simulink model "basic_dynamic_ant"  (R2022a)
settings: Solver=VariableStepAuto  StartTime=0.0  StopTime=10.0  RelTol=1e-3
values from neighbouring files (symbols this model uses):
  configSequence = [robot.Bodies{4}.Joint.PositionLimits; -robot.Bodies{7}.Joint.PositionLimits]    [ant_grasp_only.m]
  dq0 = zeros(size(q0))    [ant_grasp_only.m]
  q0 = homeConfiguration(robot)    [ant_grasp_only.m]
  widgetDimensions = [0.2 0.02 0.07]    [ant_grasp_only.m]
undefined symbols (not defined in the file or in its folder): CenterTable, Floor, LeftShelf, X, Y, Z
libraries: sm_lib x137, nesl_utility x13, robotmaniplib x3, robotcorelib x1
(part 5 of 5)

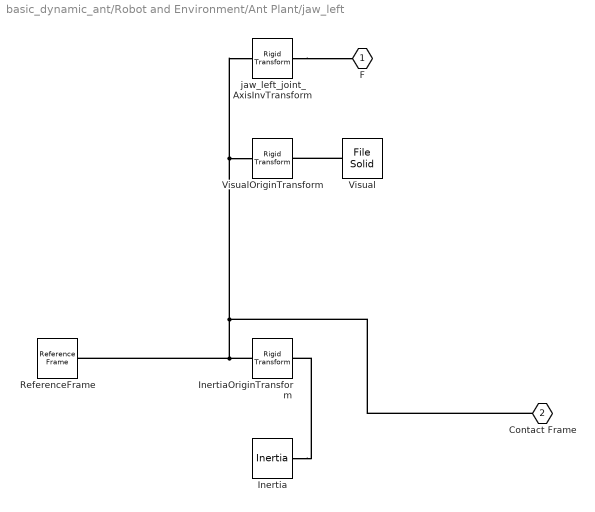
== system basic_dynamic_ant/Robot and Environment/Ant Plant/jaw_left ==
  Inertia : sm_lib/Body Elements/Inertia  InertiaType=Custom  Mass=0.01  MassUnits=kg  CenterOfMass=[0, 0, 0]  CenterOfMassUnits=m  MomentsOfInertia=[1e-06, 1e-06, 1e-06]  MomentsOfInertiaUnits=kg*m^2  ProductsOfInertia=[0, 0, 0]  ProductsOfInertiaUnits=kg*m^2  GraphicType=None  MarkerShape=Inertia  MarkerSize=20  GraphicVisPropType=SimpleVisualProperties  GraphicDiffuseColor=[0.5 0.5 0.5]  GraphicSpecularColor=[0.5 0.5 0.5 1.0]  GraphicAmbientColor=[0.15 0.15 0.15 1.0]  GraphicEmissiveColor=[0.0 0.0 0.0 1.0]  GraphicShininess=75  GraphicOpacity=1.0
  InertiaOriginTransform : sm_lib/Frames and Transforms/Rigid Transform  TranslationMethod=Cartesian  TranslationStandardOffset=0  TranslationLengthUnit=m  TranslationStandardAxis=+Z  TranslationCartesianOffset=[0, 0, 0]  TranslationROffset=0  TranslationROffsetUnits=m  TranslationZOffset=0  TranslationZOffsetUnits=m  TranslationThetaOffset=0  TranslationThetaOffsetUnits=deg  RotationMethod=RotationSequence  RotationAngleUnits=deg  RotationStandardAxis=+Z  RotationAngle=0.0  RotationArbitraryAxis=[0 0 1]  FollAlignAxisA=+X  BaseAlignAxisA=+Y  FollAlignAxisB=+Y  BaseAlignAxisB=+Z  RotationSequenceAxes=BaseAxes  RotationSequence=XYZ  RotationSequenceAngles=[0, 0, 0]  RotationSequenceAnglesUnits=rad  RotationMatrix=[1 0 0; 0 1 0; 0 0 1]
  ReferenceFrame : sm_lib/Frames and Transforms/Reference Frame
  Visual : sm_lib/Body Elements/File Solid  ExtGeomFileName=C:\Users\eroll\Documents\MATLAB\Model\ant_grasp_matlab\Simulink-Simscape-Syngrasp\ant_description\simplified_messor_mandible_left.stl  UnitType=Custom  ExtGeomFileUnits=mm  StepReaderType=HEX  ExportConvexHullGeometry=off  InertiaType=Custom  Mass=0  MassUnits=kg  CenterOfMass=[0, 0, 0]  CenterOfMassUnits=m  MomentsOfInertia=[0, 0, 0]  MomentsOfInertiaUnits=kg*m^2  ProductsOfInertia=[0, 0, 0]  ProductsOfInertiaUnits=kg*m^2  BasedOnType=DensityFromFile  Density=1000  DensityUnits=kg/m^3  DoExposeReferenceFrame=on  SerializedFrames=<Frames/>  GraphicType=FromGeometry  MarkerShape=Sphere  MarkerSize=10  GraphicVisPropType=SimpleVisualProperties  GraphicDiffuseColor=[0, 0, 0.8]  GraphicSpecularColor=[0.5 0.5 0.5 1.0]  GraphicAmbientColor=[0.15 0.15 0.15 1.0]  GraphicEmissiveColor=[0.0 0.0 0.0 1.0]  GraphicShininess=75  GraphicOpacity=1
  VisualOriginTransform : sm_lib/Frames and Transforms/Rigid Transform  TranslationMethod=Cartesian  TranslationStandardOffset=1  TranslationLengthUnit=mm  TranslationStandardAxis=+Z  TranslationCartesianOffset=[-10, -1, -17]  TranslationROffset=0  TranslationROffsetUnits=m  TranslationZOffset=0  TranslationZOffsetUnits=m  TranslationThetaOffset=0  TranslationThetaOffsetUnits=deg  RotationMethod=RotationSequence  RotationAngleUnits=deg  RotationStandardAxis=+Z  RotationAngle=0.0  RotationArbitraryAxis=[0 0 1]  FollAlignAxisA=+X  BaseAlignAxisA=+Y  FollAlignAxisB=+Y  BaseAlignAxisB=+Z  RotationSequenceAxes=BaseAxes  RotationSequence=XYZ  RotationSequenceAngles=[51,-18,-20]  RotationSequenceAnglesUnits=deg  RotationMatrix=[1 0 0; 0 1 0; 0 0 1]
  jaw_left_joint_AxisInvTransform : sm_lib/Frames and Transforms/Rigid Transform  TranslationMethod=Cartesian  TranslationStandardOffset=0  TranslationLengthUnit=m  TranslationStandardAxis=+Z  TranslationCartesianOffset=[0, 0, 0]  TranslationROffset=0  TranslationROffsetUnits=m  TranslationZOffset=0  TranslationZOffsetUnits=m  TranslationThetaOffset=0  TranslationThetaOffsetUnits=deg  RotationMethod=ArbitraryAxis  RotationAngleUnits=rad  RotationStandardAxis=+Z  RotationAngle=0  RotationArbitraryAxis=[-0, 0, 0]  FollAlignAxisA=+X  BaseAlignAxisA=+Y  FollAlignAxisB=+Y  BaseAlignAxisB=+Z  RotationSequenceAxes=FollowerAxes  RotationSequence=XYX  RotationSequenceAngles=[0 0 0]  RotationSequenceAnglesUnits=deg  RotationMatrix=[1 0 0; 0 1 0; 0 0 1]
  F : PMIOPort  Side=Left
  Contact Frame : PMIOPort  Port=2  Side=Right
  connections:
  ReferenceFrame/RConn1 -- InertiaOriginTransform/LConn1 -- jaw_left_joint_AxisInvTransform/LConn1 -- VisualOriginTransform/LConn1 -- Contact Frame/RConn1
  jaw_left_joint_AxisInvTransform/RConn1 -- F/RConn1
  Inertia/RConn1 -- InertiaOriginTransform/RConn1
  Visual/RConn1 -- VisualOriginTransform/RConn1

== system basic_dynamic_ant/Robot and Environment/Ant Plant/jaw_right ==
  Inertia : sm_lib/Body Elements/Inertia  InertiaType=Custom  Mass=0.01  MassUnits=kg  CenterOfMass=[0, 0, 0]  CenterOfMassUnits=m  MomentsOfInertia=[1e-06, 1e-06, 1e-06]  MomentsOfInertiaUnits=kg*m^2  ProductsOfInertia=[0, 0, 0]  ProductsOfInertiaUnits=kg*m^2  GraphicType=None  MarkerShape=Inertia  MarkerSize=20  GraphicVisPropType=SimpleVisualProperties  GraphicDiffuseColor=[0.5 0.5 0.5]  GraphicSpecularColor=[0.5 0.5 0.5 1.0]  GraphicAmbientColor=[0.15 0.15 0.15 1.0]  GraphicEmissiveColor=[0.0 0.0 0.0 1.0]  GraphicShininess=75  GraphicOpacity=1.0
  InertiaOriginTransform : sm_lib/Frames and Transforms/Rigid Transform  TranslationMethod=Cartesian  TranslationStandardOffset=0  TranslationLengthUnit=m  TranslationStandardAxis=+Z  TranslationCartesianOffset=[0, 0, 0]  TranslationROffset=0  TranslationROffsetUnits=m  TranslationZOffset=0  TranslationZOffsetUnits=m  TranslationThetaOffset=0  TranslationThetaOffsetUnits=deg  RotationMethod=RotationSequence  RotationAngleUnits=deg  RotationStandardAxis=+Z  RotationAngle=0.0  RotationArbitraryAxis=[0 0 1]  FollAlignAxisA=+X  BaseAlignAxisA=+Y  FollAlignAxisB=+Y  BaseAlignAxisB=+Z  RotationSequenceAxes=BaseAxes  RotationSequence=XYZ  RotationSequenceAngles=[0, 0, 0]  RotationSequenceAnglesUnits=rad  RotationMatrix=[1 0 0; 0 1 0; 0 0 1]
  ReferenceFrame : sm_lib/Frames and Transforms/Reference Frame
  Visual : sm_lib/Body Elements/File Solid  ExtGeomFileName=C:\Users\eroll\Documents\MATLAB\Model\ant_grasp_matlab\Simulink-Simscape-Syngrasp\ant_description\simplified_messor_mandible_right.stl  UnitType=Custom  ExtGeomFileUnits=mm  StepReaderType=HEX  ExportConvexHullGeometry=off  InertiaType=Custom  Mass=0  MassUnits=kg  CenterOfMass=[0, 0, 0]  CenterOfMassUnits=m  MomentsOfInertia=[0, 0, 0]  MomentsOfInertiaUnits=kg*m^2  ProductsOfInertia=[0, 0, 0]  ProductsOfInertiaUnits=kg*m^2  BasedOnType=DensityFromFile  Density=1000  DensityUnits=kg/m^3  DoExposeReferenceFrame=on  SerializedFrames=<Frames/>  GraphicType=FromGeometry  MarkerShape=Sphere  MarkerSize=10  GraphicVisPropType=SimpleVisualProperties  GraphicDiffuseColor=[0, 0, 0.8]  GraphicSpecularColor=[0.5 0.5 0.5 1.0]  GraphicAmbientColor=[0.15 0.15 0.15 1.0]  GraphicEmissiveColor=[0.0 0.0 0.0 1.0]  GraphicShininess=75  GraphicOpacity=1
  VisualOriginTransform : sm_lib/Frames and Transforms/Rigid Transform  TranslationMethod=Cartesian  TranslationStandardOffset=0  TranslationLengthUnit=mm  TranslationStandardAxis=+Z  TranslationCartesianOffset=[-10, 8, -17]  TranslationROffset=0  TranslationROffsetUnits=m  TranslationZOffset=0  TranslationZOffsetUnits=m  TranslationThetaOffset=0  TranslationThetaOffsetUnits=deg  RotationMethod=RotationSequence  RotationAngleUnits=deg  RotationStandardAxis=+Z  RotationAngle=0.0  RotationArbitraryAxis=[0 0 1]  FollAlignAxisA=+X  BaseAlignAxisA=+Y  FollAlignAxisB=+Y  BaseAlignAxisB=+Z  RotationSequenceAxes=BaseAxes  RotationSequence=XYZ  RotationSequenceAngles=[51,-18,-20]  RotationSequenceAnglesUnits=deg  RotationMatrix=[1 0 0; 0 1 0; 0 0 1]
  jaw_right_joint_AxisInvTransform : sm_lib/Frames and Transforms/Rigid Transform  TranslationMethod=Cartesian  TranslationStandardOffset=0  TranslationLengthUnit=m  TranslationStandardAxis=+Z  TranslationCartesianOffset=[0, 0, 0]  TranslationROffset=0  TranslationROffsetUnits=m  TranslationZOffset=0  TranslationZOffsetUnits=m  TranslationThetaOffset=0  TranslationThetaOffsetUnits=deg  RotationMethod=ArbitraryAxis  RotationAngleUnits=deg  RotationStandardAxis=+Z  RotationAngle=0  RotationArbitraryAxis=[-0, 0, 0]  FollAlignAxisA=+X  BaseAlignAxisA=+Y  FollAlignAxisB=+Y  BaseAlignAxisB=+Z  RotationSequenceAxes=FollowerAxes  RotationSequence=XYX  RotationSequenceAngles=[0 0 0]  RotationSequenceAnglesUnits=deg  RotationMatrix=[1 0 0; 0 1 0; 0 0 1]
  F : PMIOPort  Side=Left
  Contact Frame : PMIOPort  Port=2  Side=Right
  connections:
  ReferenceFrame/RConn1 -- InertiaOriginTransform/LConn1 -- jaw_right_joint_AxisInvTransform/LConn1 -- VisualOriginTransform/LConn1 -- Contact Frame/RConn1
  Inertia/RConn1 -- InertiaOriginTransform/RConn1
  Visual/RConn1 -- VisualOriginTransform/RConn1
  jaw_right_joint_AxisInvTransform/RConn1 -- F/RConn1

== matlab function basic_dynamic_ant/Task & Trajectory Scheduler ==
  settings: updateMethod=DISCRETE
  data: inputTime input; configSequence input; state output; closeGripper output; robotConfig input; t output; wpts output; gripperStateReached input
function [state, closeGripper, t, wpts] = commandLogic(inputTime, configSequence, robotConfig, gripperStateReached)

persistent motionState
persistent resetTimeValue

% Set some variables
posTgtThreshold = 0.015;

% Initialize persistent variables
if isempty(motionState)
    motionState = 1;
end
if isempty(resetTimeValue)
    resetTimeValue = 0;
end

% Output the state and time
state = motionState;
t = inputTime - resetTimeValue;

% Initialize outputs to starting state
wpts = configSequence;
closeGripper = false;

switch motionState
    case 1
        % Open the gripper
        wpts = [robotConfig configSequence(:,2)];
        
        closeGripper = false;
    case 2
        % Close the gripper
        wpts = [robotConfig configSequence(:,1)];
        
        closeGripper = true;
end
   
% Get the current status
trajEndConfigReached = endStateReached(robotConfig, wpts, posTgtThreshold);

% Advance the state and reset time as needed
if trajEndConfigReached && gripperStateReached
    % Advance the state and reset the time
    motionState = mod(motionState, 2) + 1;
    resetTimeValue = inputTime;
end

end

function isReached = endStateReached(config, wpts, tgtThreshold)
    
    % Initialize output
    isReached = false;

    %Extract the arm that matters and then ignore the gripper position
    armConfig = config;
    armTarget = wpts(:,2);
    
    % Check if the arm states match the target waypoints
    diffWpts = zeros(2,1);
    diffWpts(:,:) = abs(armConfig - armTarget);
    errorStatus = diffWpts < tgtThreshold;
    if all(errorStatus)
        isReached = true;
    end
end

== matlab function basic_dynamic_ant/Robot and Environment/Gripper Sensor/Gripper Logic ==
  data: closeGripperCmd input; gripperPos input; isStateReached output; isGrippingObj input
function isStateReached = isGripperStateReached(closeGripperCmd, gripperPos, isGrippingObj)

    % Define key values
    posTgtThreshold = 0.01;
    openValue = 0.5;
    closeValue = 0;
    
    % Determine if the state is reached based on two cases: when the
    % command is to close the gripper, and when the command is to open the
    % gripper
    if closeGripperCmd        
        % When the gripper is closed, the state is reached if either the
        % gripper is closed all the way, or the gripper has a firm grasp of
        % the object to be gripped
        
        isPosStateReached = isGripperTargetPositionReached(gripperPos, closeValue, posTgtThreshold);
        isStateReached = (isPosStateReached || isGrippingObj);
    else
        % When the gripper is opened, the state is reached only if the
        % gripper reaches its target fully open position
        isStateReached = isGripperTargetPositionReached(gripperPos, openValue, posTgtThreshold);
    end    
end

function isReached = isGripperTargetPositionReached(gripperPos, gripperTarget, tgtThreshold)
%isGripperTargetPositionReached Returns TRUE if gripper target position is reached

    isReached = false;

    % Check if the gripper joints have reached their open target
    diffWpts = abs(gripperPos - [gripperTarget; gripperTarget]);
    posErrorStatus = diffWpts < tgtThreshold;
    
    if all(posErrorStatus)
        isReached = true;
    end
end

== matlab function basic_dynamic_ant/Robot and Environment/Widget to Environment Contact/MATLAB Function ==
  data: objectTransform input; collisionObjectArray output; vertices input
function collisionObjectArray = object2CollisionSpheres(objectTransform, vertices)

collisionObjectArray = u;
